simulink model "dcpa"  (Simulink 3.00)
settings: Solver=ode45  SolverMode=SingleTasking  StartTime=0.0  StopTime=20  MaxStep=.010  RelTol=1e-3  AbsTol=1e-3
settings Model: TimeSaveName=t  SaveOutput=off

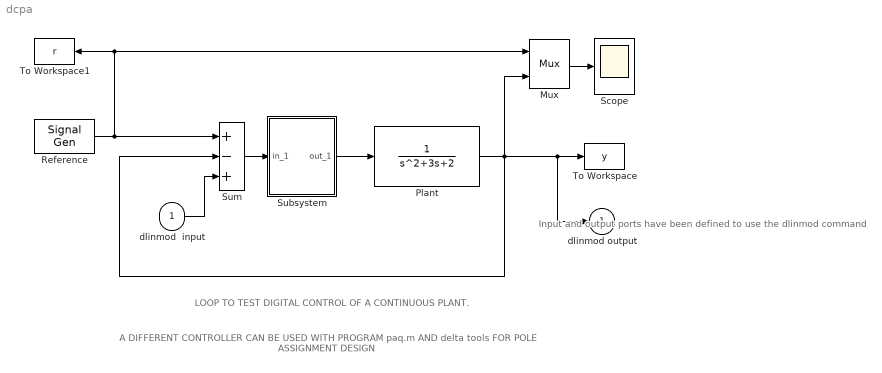
== system dcpa ==
  note: LOOP TO TEST DIGITAL CONTROL OF A CONTINUOUS PLANT.
  note: A DIFFERENT CONTROLLER CAN BE USED
      | WITH  PROGRAM paq.m AND delta tools FOR POLE ASSIGNMENT DESIGN
  note: Input and output ports
      | have been defined to
      | use the dlinmod command
  dlinmod  input : Inport  Port=1  PortWidth=-1  SampleTime=-1  DataType=auto
      settings: SignalType=auto
  Mux : Mux  Inputs=2
      settings: DisplayOption=none
  Plant : TransferFcn  Numerator=[1]  Denominator="[1 3  2]"
  Reference : SignalGenerator  WaveForm=square  Amplitude=1.000000  Frequency=0.315000  Units=rad/sec
  Scope : Scope
      settings: TickLabels=on  TimeRange=20.000000  YMin=-2  YMax=2  SaveToWorkspace=off  SaveName=ScopeData  DataFormat=Matrix
  Subsystem : Subsystem  mask(Digital controller){@1=[29.12 -48.25  20], @2=[1  -1.21  0.21], @3=0.1}
      mask prompts: @1 "numerator:"; @2 "denominator:"; @3 "sampling period:"
      mask help: Digital controller
      mask init:
      | ncq=@1;dcq=@2;T=@3;
      mask Display: disp('C(z)')
  Sum : Sum  Inputs=+-+  SaturateOnIntegerOverflow=on
  To Workspace : ToWorkspace  VariableName=y  SampleTime=0  SaveFormat=Matrix
      settings: Buffer=10000
  To Workspace1 : ToWorkspace  VariableName=r  SampleTime=0  SaveFormat=Matrix
      settings: Buffer=10000
  dlinmod output : Outport  Port=1  InitialOutput=0
  wires:
  Subsystem/1(out_1) -> Plant/1
  Sum/1 -> Subsystem/1(in_1)
  Mux/1 -> Scope/1
  dlinmod  input/1 -> Sum/3
  Reference/1 -> Sum/1, Mux/1, To Workspace1/1
  Plant/1 -> To Workspace/1, dlinmod output/1, Sum/2, Mux/2

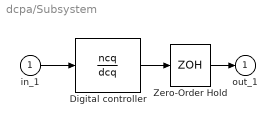
== system dcpa/Subsystem ==
  in_1 : Inport  Port=1  PortWidth=-1  SampleTime=-1  DataType=auto
      settings: SignalType=auto
  Digital controller : DiscreteTransferFcn  Numerator=ncq  Denominator=dcq  SampleTime=T
  Zero-Order Hold : ZeroOrderHold  SampleTime=T
  out_1 : Outport  Port=1  InitialOutput=0
  wires:
  Digital controller/1 -> Zero-Order Hold/1
  in_1/1 -> Digital controller/1
  Zero-Order Hold/1 -> out_1/1
